simulink model "messageModel"  (R2024b)
settings: configuration reference "model_cfg" (kept outside this file)
model workspace (MATLAB code in the model file):
  | cmdLim = Simulink.Parameter;
  | cmdLim.Value = 15;
  | cmdLim.Description = 'Limit for controlling the maximum surface command angle.';
  | cmdLim.Min = 0;
  | cmdLim.Max = 90;
  | cmdLim.DocUnits = 'deg';
  | 
  | dispGain = Simulink.Parameter;
  | dispGain.Value = 0.75;
  | dispGain.Description = 'Gain applied to the displacement error.';
  | dispGain.Min = 0;
  | dispGain.Max = [];
  | dispGain.DocUnits = 'deg/sec/deg';
  | 
  | dispLim = Simulink.Parameter;
  | dispLim.Value = 30;
  | dispLim.Description = 'Limit for controlling the maximum commanded angle.';
  | dispLim.Min = 0;
  | dispLim.Max = 180;
  | dispLim.DocUnits = 'deg';
  | 
  | intGain = Simulink.Parameter;
  | intGain.Value = 0.5;
  | intGain.Description = 'Gain applied to the integral error.';
  | intGain.Min = 0;
  | intGain.Max = [];
  | intGain.DocUnits = 'deg/sec/deg/sec';
  | 
  | intLim = Simulink.Parameter;
  | intLim.Value = 5;
  | intLim.Description = 'Limit for controlling the maximum commanded angle.';
  | intLim.Min = 0;
  | intLim.Max = 90;
  | intLim.DocUnits = 'deg';
  | 
  | rateGain = Simulink.Parameter;
  | rateGain.Value = 2;
  | rateGain.Description = 'Gain applied to the rate error.';
  | rateGain.Min = 0;
  | rateGain.Max = [];
  | rateGain.DocUnits = 'deg/deg/sec';
  | 
  | rateLim = Simulink.Parameter;
  | rateLim.Value = 6;
  | rateLim.Description = 'Limit for controlling the maximum commanded angle.';
  | rateLim.Min = 0;
  | rateLim.Max = 180;
  | rateLim.DocUnits = 'deg/sec';
  | 
  | hdgGain = Simulink.Parameter;
  | hdgGain.Value = 0.015;
settings Model: RequirementInfo={} %GIDa_fe9045fd_0412_4b6e_8206_617cc20e6fde  Creator=nabilekhoury  LastModifiedBy=nabilekhoury
settings ConfigSetRef: SourceName=model_cfg  SourceLocation=Base Workspace

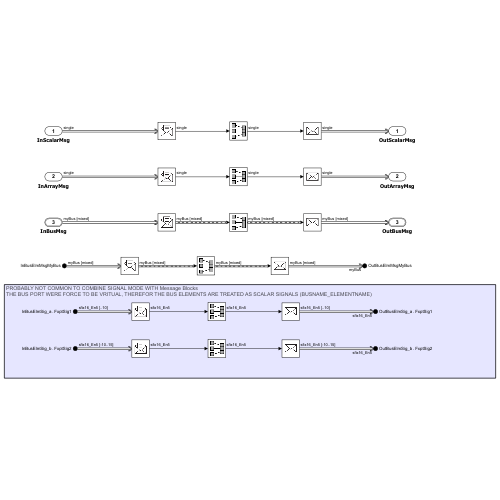
[thumbnail: Simulink's stored preview of the top-level diagram]
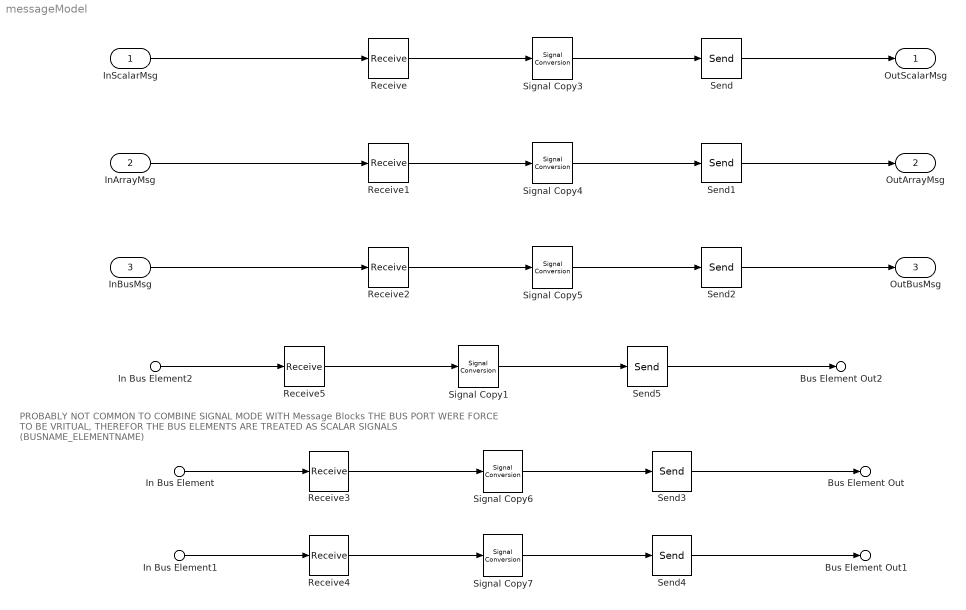
== system messageModel ==
  note: PROBABLY NOT COMMON TO COMBINE SIGNAL MODE WITH Message Blocks
      | THE BUS PORT WERE FORCE TO BE VRITUAL, THEREFOR THE BUS ELEMENTS ARE TREATED AS SCALAR SIGNALS (BUSNAME_ELEMENTNAME)
  InScalarMsg : Inport  OutputPortMessageModes=m  OutDataTypeStr=single
  InArrayMsg : Inport  OutputPortMessageModes=m  Port=2  OutDataTypeStr=single  PortDimensions=2
  InBusMsg : Inport  OutputPortMessageModes=m  Port=3  OutDataTypeStr=Bus: myBus  BusOutputAsStruct=on
  In Bus Element2 : Inport  Port=4  PortName=InBusElmMsgMyBus
  In Bus Element : Inport  Port=5  PortName=InBusElmSig_a  Element=FxptSig1
  In Bus Element1 : Inport  Port=6  PortName=InBusElmSig_b  Element=FxptSig2
  Receive{,1..5} (6 alike) : Receive  InputPortMessageModes=m  UseInternalQueue=off  QueueOverwriting=on  QueueLength=1  QueueType=LIFO
  Send{,1..5} (6 alike) : Send  OutputPortMessageModes=m
  Signal Copy{1,3..7} (6 alike) : SignalConversion  OverrideOpt=off
  OutScalarMsg : Outport  InputPortMessageModes=m  VectorParamsAs1DForOutWhenUnconnected=off
  OutArrayMsg : Outport  InputPortMessageModes=m  Port=2  PortDimensions=2  VectorParamsAs1DForOutWhenUnconnected=off
  OutBusMsg : Outport  InputPortMessageModes=m  Port=3  OutDataTypeStr=Bus: myBus  VectorParamsAs1DForOutWhenUnconnected=off  BusOutputAsStruct=on
  Bus Element Out2 : Outport  InputPortMessageModes=m  Port=4  PortName=OutBusElmMsgMyBus
  Bus Element Out : Outport  InputPortMessageModes=m  Port=5  PortName=OutBusElmSig_a  Element=FxptSig1
  Bus Element Out1 : Outport  InputPortMessageModes=m  Port=6  PortName=OutBusElmSig_b  Element=FxptSig2
  wires:
  InScalarMsg/1 -> Receive/1
  InArrayMsg/1 -> Receive1/1
  InBusMsg/1 -> Receive2/1
  Receive2/1 -> Signal Copy5/1
  Signal Copy3/1 -> Send/1
  Signal Copy4/1 -> Send1/1
  Signal Copy5/1 -> Send2/1
  In Bus Element/1 -> Receive3/1
  Signal Copy6/1 -> Send3/1
  Receive/1 -> Signal Copy3/1
  Receive1/1 -> Signal Copy4/1
  Signal Copy7/1 -> Send4/1
  In Bus Element1/1 -> Receive4/1
  Send/1 -> OutScalarMsg/1
  Receive3/1 -> Signal Copy6/1
  Receive4/1 -> Signal Copy7/1
  Send1/1 -> OutArrayMsg/1
  Send2/1 -> OutBusMsg/1
  Send3/1 -> Bus Element Out/1
  Send4/1 -> Bus Element Out1/1
  Send5/1 -> Bus Element Out2/1
  Receive5/1 -> Signal Copy1/1
  In Bus Element2/1 -> Receive5/1
  Signal Copy1/1 -> Send5/1
